simulink model "SimulinkModel_hquad_lin_yaw"  (Simulink 7.6)
settings: Solver=ode45  StartTime=0.0  StopTime=10.0  RelTol=1e-3
libraries: Hqaud_model_LIB_SI x1
settings Model: Creator=andi  LastModifiedBy=burrimi
settings DebuggingCC: StrictBusMsg=Warning

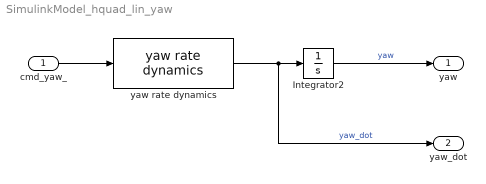
== system SimulinkModel_hquad_lin_yaw ==
  "cmd_yaw_  " : Inport
  Integrator2 : Integrator
  yaw rate dynamics : Hqaud_model_LIB_SI/yaw rate dynamics    SystemSampleTime=-1
  yaw : Outport
  yaw_dot : Outport  Port=2
  wires:
  "cmd_yaw_  "/1 -> yaw rate dynamics/1
  Integrator2/1 -> yaw/1  "yaw"
  yaw rate dynamics/1 -> Integrator2/1, yaw_dot/1  "yaw_dot"
